simulink model "crazyflie_2015a"  (R2015a)
settings: Solver=ode3  StartTime=0.0  StopTime=30  FixedStep=1/500  MinStep=1e-4  RelTol=1e-3
undefined symbols (not defined in the file): A, B, C, D
libraries: simulink x2
settings Model: NumberOfSteps=250  CovModelRefEnable=off  Creator=mattcollins  LastModifiedBy=mattcollins
settings DataIOCC: SaveFormat=Dataset
settings HardwareCC: ProdBitPerPointer=64  ProdLargestAtomicFloat=Float  ProdIntDivRoundTo=Zero  ProdEndianess=LittleEndian  ProdHWDeviceType=Specified
settings GRTTargetCC: GeneratePreprocessorConditionals=Use local settings

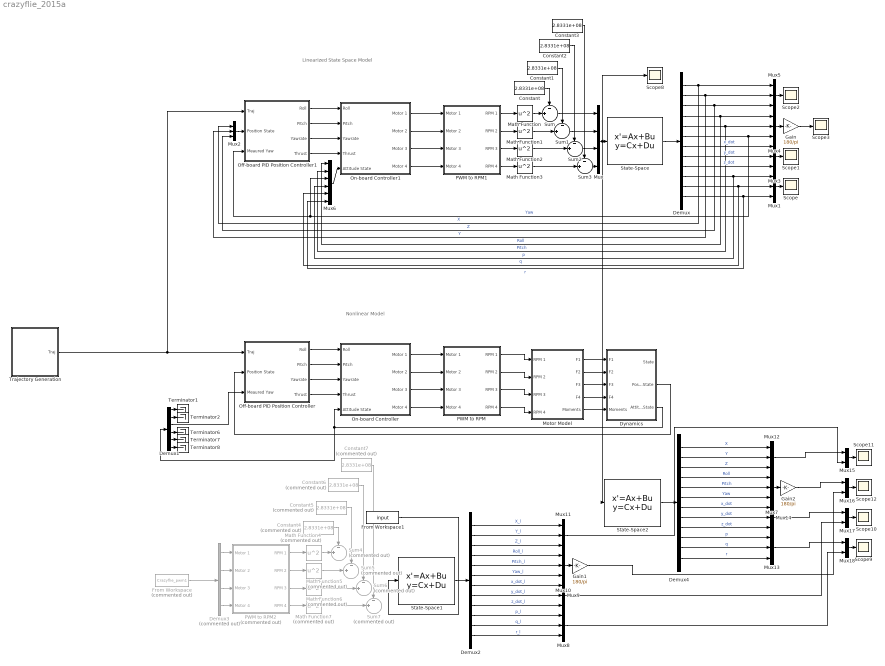
== system crazyflie_2015a ==
  note: Nonlinear Model
  note: Linearized State Space Model
  Constant{,1..3} (4 alike) : Constant  Value=2.8331e+08
  Constant{4..7} (4 alike) : Constant  Commented=on  Value=2.8331e+08
  Demux : Demux  Outputs=12
  Demux1 : Demux  Outputs=6
  Demux2 : Demux  Outputs=12
  Demux3 : Demux  Commented=on
  Demux4 : Demux  Outputs=12
  Dynamics : Subsystem
  From Workspace : FromWorkspace  Commented=on  VariableName=Crazyflie_pwm1  SampleTime=1/500
  From Workspace1 : FromWorkspace  VariableName=input
  Gain : Gain  Gain=180/pi
  Gain1 : Gain  Gain=180/pi
  Gain2 : Gain  Gain=180/pi
  Math Function{,1..3} (4 alike) : Math  Operator=square  SaturateOnIntegerOverflow=on
  Math Function{4..7} (4 alike) : Math  Commented=on  Operator=square  SaturateOnIntegerOverflow=on
  Motor Model : Subsystem
  Mux : Mux
  Mux{1..5,7..14} (13 alike) : Mux  Inputs=3
  Mux{15..18} (4 alike) : Mux  Inputs=2
  Mux6 : Mux  Inputs=6
  Off-board PID Position Controller : Subsystem
  Off-board PID Position Controller1 : Subsystem
  On-board Controller : Subsystem
  On-board Controller1 : Subsystem
  PWM to RPM : Subsystem
  PWM to RPM1 : Subsystem
  PWM to RPM2 : Subsystem  Commented=on
  Scope{,1..3,8..12} (9 alike) : Scope
      Scope settings: TimeRange=auto  ShowLegends=on  MaxDataPoints=5000  SaveToWorkspace=off  YMin=-0.989  YMax=2.74983  SampleTime=-1
      Scope1 settings: TimeRange=auto  ShowLegends=on  MaxDataPoints=5000  SaveToWorkspace=off  SaveName=ScopeData2  YMin=-0.02898  YMax=0.02839  SampleTime=-1
      Scope10 settings: TimeRange=auto  ShowLegends=on  MaxDataPoints=5000  SaveToWorkspace=off  YMin=-5  YMax=5  SampleTime=-1
      Scope11 settings: TimeRange=auto  ShowLegends=on  MaxDataPoints=5000  SaveToWorkspace=off  SaveName=ScopeData2  YMin=-3.50437  YMax=3  SampleTime=-1  DataFormat=Array
      Scope12 settings: TimeRange=auto  ShowLegends=on  MaxDataPoints=5000  SaveToWorkspace=off  SaveName=ScopeData3  YMin=-8.76362  YMax=25  SampleTime=-1  DataFormat=Array
      Scope2 settings: TimeRange=auto  ShowLegends=on  MaxDataPoints=5000  SaveName=Pos_Lin  YMin=-0.86443  YMax=1.76271  SampleTime=-1  DataFormat=Array
      Scope3 settings: TimeRange=auto  ShowLegends=on  MaxDataPoints=5000  SaveName=Att_Lin  YMin=-9.06868  YMax=18.0573  SampleTime=-1  DataFormat=Array
      Scope8 settings: TimeRange=auto  ShowLegends=on  MaxDataPoints=5000  SaveName=input  YMin=-405553.36028  YMax=400152.57445  SampleTime=-1  DataFormat=Array
      Scope9 settings: TimeRange=auto  ShowLegends=on  MaxDataPoints=5000  SaveToWorkspace=off  SaveName=ScopeData4  YMin=-0.989  YMax=2.74983  SampleTime=-1
  State-Space : StateSpace  A=A  B=B  C=C  D=D  X0=[0;0;0;0;0;0;0;0;0;0;0;0]
  State-Space1 : StateSpace  A=A  B=B  C=C  D=D  X0=[0;0;0;0;0;0;0;0;0;0;0;0]
  State-Space2 : StateSpace  A=A  B=B  C=C  D=D  X0=[0;0;0;0;0;0;0;0;0;0;0;0]
  Sum{,1..3} (4 alike) : Sum  Inputs=-|+||
  Sum{4..7} (4 alike) : Sum  Commented=on  Inputs=-|+||
  Terminator{1..2,6..8} (5 alike) : Terminator
  Trajectory Generation : Subsystem
  wires:
  On-board Controller/1(Motor 1) -> PWM to RPM/1(Motor 1)
  On-board Controller/2(Motor 2) -> PWM to RPM/2(Motor 2)
  On-board Controller/3(Motor 3) -> PWM to RPM/3(Motor 3)
  On-board Controller/4(Motor 4) -> PWM to RPM/4(Motor 4)
  PWM to RPM/1(RPM 1) -> Motor Model/1(RPM 1)
  PWM to RPM/2(RPM 2) -> Motor Model/2(RPM 2)
  PWM to RPM/3(RPM 3) -> Motor Model/3(RPM 3)
  PWM to RPM/4(RPM 4) -> Motor Model/4(RPM 4)
  Motor Model/1(F1) -> Dynamics/1(F1)
  Dynamics/3(Attitude State) -> On-board Controller/5(Attitude State), Demux1/1
  Off-board PID Position Controller/1(Roll) -> On-board Controller/1(Roll)
  Off-board PID Position Controller/2(Pitch) -> On-board Controller/2(Pitch)
  Off-board PID Position Controller/3(Yawrate) -> On-board Controller/3(Yawrate)
  Off-board PID Position Controller/4(Thrust) -> On-board Controller/4(Thrust)
  Dynamics/2(Position State) -> Off-board PID Position Controller/2(Position State)
  Motor Model/2(F2) -> Dynamics/2(F2)
  Motor Model/3(F3) -> Dynamics/3(F3)
  Motor Model/4(F4) -> Dynamics/4(F4)
  Motor Model/5(Moments) -> Dynamics/5(Moments)
  Demux1/3 -> Off-board PID Position Controller/3(Meaured Yaw)
  Demux1/1 -> Terminator1/1
  Demux1/2 -> Terminator2/1
  Demux1/4 -> Terminator6/1
  Demux1/5 -> Terminator7/1
  Demux1/6 -> Terminator8/1
  State-Space/1 -> Demux/1
  Demux/10 -> Mux6/4, Mux1/1  "p"
  Demux/11 -> Mux6/5, Mux1/2  "q"
  Demux/12 -> Mux6/6, Mux1/3  "r"
  Mux1/1 -> Scope/1
  Mux3/1 -> Scope1/1
  Demux/7 -> Mux3/1  "x_dot"
  Demux/8 -> Mux3/2  "y_dot"
  Demux/9 -> Mux3/3  "z_dot"
  Demux/4 -> Mux6/1, Mux4/1  "Roll"
  Demux/5 -> Mux6/2, Mux4/2  "Pitch"
  Demux/6 -> Mux6/3, Off-board PID Position Controller1/3(Meaured Yaw), Mux4/3  "Yaw"
  Demux/1 -> Mux2/1, Mux5/1  "X"
  Demux/2 -> Mux2/2, Mux5/2  "Y"
  Demux/3 -> Mux2/3, Mux5/3  "Z"
  Mux4/1 -> Gain/1
  Mux5/1 -> Scope2/1
  PWM to RPM1/1(RPM 1) -> Math Function/1
  PWM to RPM1/2(RPM 2) -> Math Function1/1
  PWM to RPM1/3(RPM 3) -> Math Function2/1
  PWM to RPM1/4(RPM 4) -> Math Function3/1
  On-board Controller1/2(Motor 2) -> PWM to RPM1/2(Motor 2)
  On-board Controller1/3(Motor 3) -> PWM to RPM1/3(Motor 3)
  On-board Controller1/4(Motor 4) -> PWM to RPM1/4(Motor 4)
  Off-board PID Position Controller1/1(Roll) -> On-board Controller1/1(Roll)
  Off-board PID Position Controller1/2(Pitch) -> On-board Controller1/2(Pitch)
  Off-board PID Position Controller1/3(Yawrate) -> On-board Controller1/3(Yawrate)
  Off-board PID Position Controller1/4(Thrust) -> On-board Controller1/4(Thrust)
  Trajectory Generation/1(Traj) -> Off-board PID Position Controller1/1(Traj), Off-board PID Position Controller/1(Traj)
  Mux2/1 -> Off-board PID Position Controller1/2(Position State)
  Mux6/1 -> On-board Controller1/5(Attitude State)
  Gain/1 -> Scope3/1
  Sum/1 -> Mux/1
  Math Function/1 -> Sum/2
  Constant/1 -> Sum/1
  Math Function3/1 -> Sum3/2
  Math Function2/1 -> Sum2/2
  Sum1/1 -> Mux/2
  Math Function1/1 -> Sum1/2
  Sum2/1 -> Mux/3
  Constant1/1 -> Sum1/1
  Constant2/1 -> Sum2/1
  Constant3/1 -> Sum3/1
  State-Space1/1 -> Demux2/1
  Demux2/10 -> Mux8/1  "p_l"
  Demux2/11 -> Mux8/2  "q_l"
  Demux2/12 -> Mux8/3  "r_l"
  Mux8/1 -> Mux18/2
  Mux9/1 -> Mux17/2
  Demux2/7 -> Mux9/1  "x_dot_l"
  Demux2/8 -> Mux9/2  "y_dot_l"
  Demux2/9 -> Mux9/3  "z_dot_l"
  Demux2/4 -> Mux10/1  "Roll_l"
  Demux2/5 -> Mux10/2  "Pitch_l"
  Demux2/6 -> Mux10/3  "Yaw_l"
  Demux2/1 -> Mux11/1  "X_l"
  Demux2/2 -> Mux11/2  "Y_l"
  Demux2/3 -> Mux11/3  "Z_l"
  Mux10/1 -> Gain1/1
  Mux11/1 -> Mux15/2
  PWM to RPM2/1(RPM 1) -> Math Function4/1
  PWM to RPM2/2(RPM 2) -> Math Function5/1
  PWM to RPM2/3(RPM 3) -> Math Function6/1
  PWM to RPM2/4(RPM 4) -> Math Function7/1
  Gain1/1 -> Mux16/2
  Math Function4/1 -> Sum4/2
  Constant4/1 -> Sum4/1
  Math Function7/1 -> Sum7/2
  Math Function6/1 -> Sum6/2
  Math Function5/1 -> Sum5/2
  Constant5/1 -> Sum5/1
  Constant6/1 -> Sum6/1
  Constant7/1 -> Sum7/1
  Demux3/1 -> PWM to RPM2/1(Motor 1)
  Demux3/2 -> PWM to RPM2/2(Motor 2)
  Demux3/3 -> PWM to RPM2/3(Motor 3)
  Demux3/4 -> PWM to RPM2/4(Motor 4)
  From Workspace/1 -> Demux3/1
  Sum3/1 -> Mux/4
  From Workspace1/1 -> State-Space1/1
  State-Space2/1 -> Demux4/1
  Demux4/10 -> Mux13/1  "p"
  Demux4/11 -> Mux13/2  "q"
  Demux4/12 -> Mux13/3  "r"
  Demux4/7 -> Mux14/1  "x_dot"
  Demux4/8 -> Mux14/2  "y_dot"
  Demux4/9 -> Mux14/3  "z_dot"
  Demux4/4 -> Mux7/1  "Roll"
  Demux4/5 -> Mux7/2  "Pitch"
  Demux4/6 -> Mux7/3  "Yaw"
  Demux4/1 -> Mux12/1  "X"
  Demux4/2 -> Mux12/2  "Y"
  Demux4/3 -> Mux12/3  "Z"
  Mux7/1 -> Gain2/1
  Mux/1 -> Scope8/1, State-Space2/1, State-Space/1
  Mux15/1 -> Scope11/1
  Mux16/1 -> Scope12/1
  Mux17/1 -> Scope10/1
  Mux18/1 -> Scope9/1
  Mux12/1 -> Mux15/1
  Gain2/1 -> Mux16/1
  Mux14/1 -> Mux17/1
  Mux13/1 -> Mux18/1
  On-board Controller1/1(Motor 1) -> PWM to RPM1/1(Motor 1)

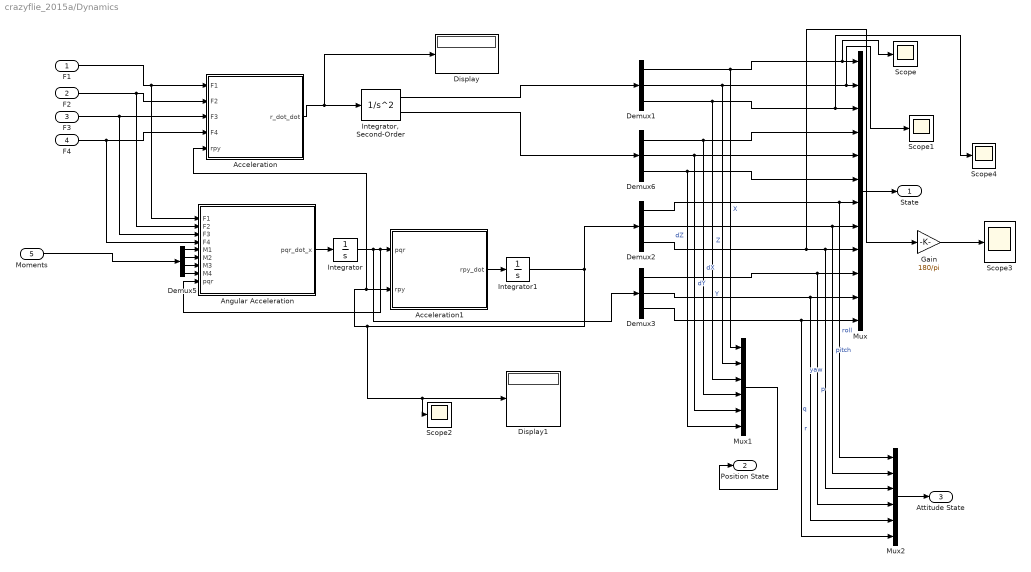
== system crazyflie_2015a/Dynamics ==
  F1 : Inport
  F2 : Inport  Port=2
  F3 : Inport  Port=3
  F4 : Inport  Port=4
  Moments : Inport  Port=5
  Acceleration : MATLAB Function  TreatAsAtomicUnit=on
      settings: PermitHierarchicalResolution=ParametersOnly
  Acceleration1 : MATLAB Function  TreatAsAtomicUnit=on
      settings: PermitHierarchicalResolution=ParametersOnly
  Angular Acceleration : MATLAB Function  TreatAsAtomicUnit=on
      settings: PermitHierarchicalResolution=ParametersOnly
  Demux{1..3,6} (4 alike) : Demux  Outputs=3
  Demux5 : Demux
  Display : Display
  Display1 : Display
  Gain : Gain  Gain=180/pi
  Integrator : Integrator  InitialCondition=[0;0;0]
  "Integrator, Second-Order" : SecondOrderIntegrator  ICX=[0;0;0]  LimitX=on  UpperLimitX=[inf,inf,inf]  LowerLimitX=[-inf,-inf,0]  StateNameX=['x', 'y', 'z']  ICDXDT=[0;0;0]  LimitDXDT=on  UpperLimitDXDT=Inf  LowerLimitDXDT=-Inf  StateNameDXDT=['dx', 'dy', 'dz']
  Integrator1 : Integrator  InitialCondition=[0;0;0]
  Mux : Mux  Inputs=12
  Mux1 : Mux  Inputs=6
  Mux2 : Mux  Inputs=6
  Scope{,1..4} (5 alike) : Scope
      Scope settings: TimeRange=auto  MaxDataPoints=5000  SaveName=x_pos  YMin=-0.15977  YMax=1.43792  SampleTime=-1  DataFormat=Array
      Scope1 settings: TimeRange=auto  MaxDataPoints=5000  SaveName=y_pos  YMin=-0.15994  YMax=1.43948  SampleTime=-1  DataFormat=Array
      Scope2 settings: TimeRange=auto  MaxDataPoints=5000  SaveToWorkspace=off  YMin=-0.00075  YMax=0.00059  SampleTime=-1
      Scope3 settings: TimeRange=auto  MaxDataPoints=5000  SaveName=yaw_pos  YMin=-7.58141  YMax=67.89856  SampleTime=-1  DataFormat=Array
      Scope4 settings: TimeRange=auto  MaxDataPoints=5000  SaveName=z_pos  YMin=0.00000  YMax=1.5  SampleTime=-1  DataFormat=Array
  State : Outport
  Position State : Outport  Port=2
  Attitude State : Outport  Port=3
  wires:
  Demux2/1 -> Mux2/1, Mux/7  "roll"
  Demux2/2 -> Mux2/2, Mux/8  "pitch"
  Demux2/3 -> Gain/1, Mux2/3, Mux/9  "yaw"
  Demux3/1 -> Mux2/4, Mux/10  "p"
  Demux3/2 -> Mux2/5, Mux/11  "q"
  Demux3/3 -> Mux2/6, Mux/12  "r"
  Mux/1 -> State/1
  Mux1/1 -> Position State/1
  Mux2/1 -> Attitude State/1
  Demux5/1 -> Angular Acceleration/5(M1)
  Demux5/2 -> Angular Acceleration/6(M2)
  Demux5/3 -> Angular Acceleration/7(M3)
  Demux5/4 -> Angular Acceleration/8(M4)
  Angular Acceleration/1(pqr_dot_x) -> Integrator/1
  Integrator/1 -> Demux3/1, Angular Acceleration/9(pqr), Acceleration1/1(pqr)
  Acceleration1/1(rpy_dot) -> Integrator1/1
  Integrator1/1 -> Demux2/1, Scope2/1, Display1/1, Acceleration/5(rpy), Acceleration1/2(rpy)
  Acceleration/1(r_dot_dot) -> Display/1, "Integrator, Second-Order"/1
  "Integrator, Second-Order"/1 -> Demux1/1
  "Integrator, Second-Order"/2 -> Demux6/1
  Demux1/1 -> Mux1/1, Scope/1, Mux/1  "X"
  Demux1/2 -> Mux1/2, Scope1/1, Mux/2  "Y"
  Demux1/3 -> Mux1/3, Scope4/1, Mux/3  "Z"
  Demux6/1 -> Mux1/4, Mux/4  "dX"
  Demux6/2 -> Mux1/5, Mux/5  "dY"
  Demux6/3 -> Mux1/6, Mux/6  "dZ"
  Moments/1 -> Demux5/1
  F2/1 -> Angular Acceleration/2(F2), Acceleration/2(F2)
  F3/1 -> Angular Acceleration/3(F3), Acceleration/3(F3)
  F4/1 -> Angular Acceleration/4(F4), Acceleration/4(F4)
  F1/1 -> Angular Acceleration/1(F1), Acceleration/1(F1)
  Gain/1 -> Scope3/1

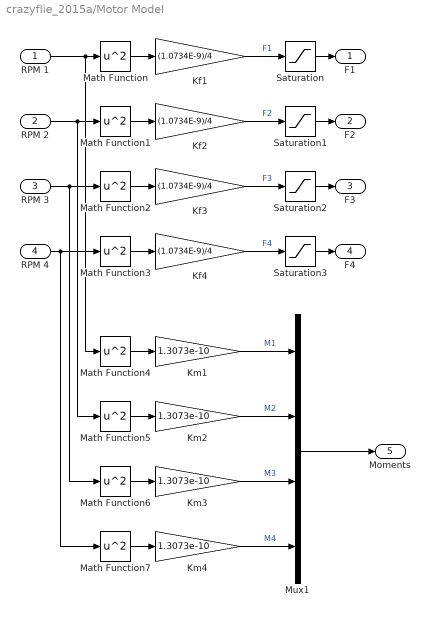
== system crazyflie_2015a/Motor Model ==
  RPM 1 : Inport
  RPM 2 : Inport  Port=2
  RPM 3 : Inport  Port=3
  RPM 4 : Inport  Port=4
  Kf{1..4} (4 alike) : Gain  Gain=(1.0734E-9)/4
  Km{1..4} (4 alike) : Gain  Gain=1.3073e-10
  Math Function{,1..7} (8 alike) : Math  Operator=square  SaturateOnIntegerOverflow=on
  Mux1 : Mux
  Saturation{,1..3} (4 alike) : Saturate  UpperLimit=.2  LowerLimit=0
  F1 : Outport
  F2 : Outport  Port=2
  F3 : Outport  Port=3
  F4 : Outport  Port=4
  Moments : Outport  Port=5
  wires:
  RPM 4/1 -> Math Function7/1, Math Function3/1
  RPM 3/1 -> Math Function6/1, Math Function2/1
  RPM 2/1 -> Math Function5/1, Math Function1/1
  RPM 1/1 -> Math Function4/1, Math Function/1
  Math Function/1 -> Kf1/1
  Math Function1/1 -> Kf2/1
  Math Function2/1 -> Kf3/1
  Math Function3/1 -> Kf4/1
  Kf3/1 -> Saturation2/1  "F3"
  Math Function4/1 -> Km1/1
  Math Function5/1 -> Km2/1
  Math Function6/1 -> Km3/1
  Math Function7/1 -> Km4/1
  Km4/1 -> Mux1/4  "M4"
  Km3/1 -> Mux1/3  "M3"
  Km2/1 -> Mux1/2  "M2"
  Km1/1 -> Mux1/1  "M1"
  Mux1/1 -> Moments/1
  Kf2/1 -> Saturation1/1  "F2"
  Kf1/1 -> Saturation/1  "F1"
  Kf4/1 -> Saturation3/1  "F4"
  Saturation/1 -> F1/1
  Saturation1/1 -> F2/1
  Saturation2/1 -> F3/1
  Saturation3/1 -> F4/1

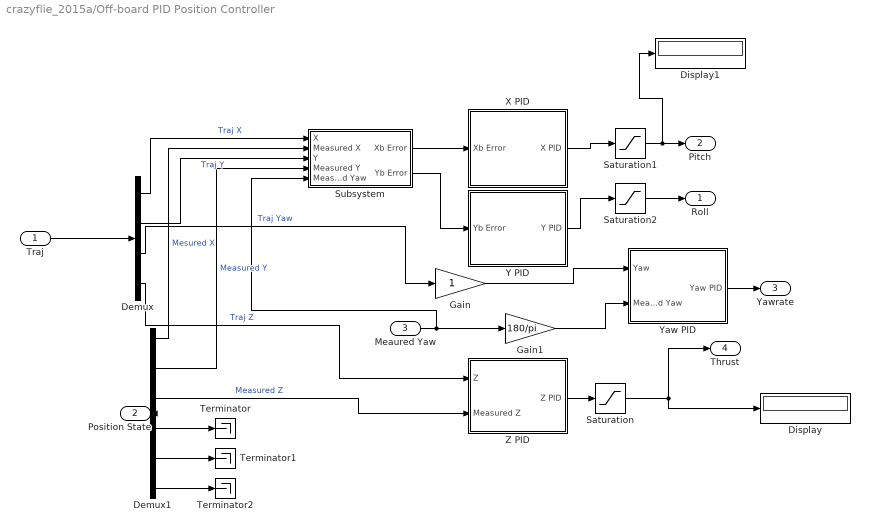
== system crazyflie_2015a/Off-board PID Position Controller ==
  Traj : Inport
  Position State : Inport  Port=2
  Meaured Yaw : Inport  Port=3
  Demux : Demux
  Demux1 : Demux  Outputs=6
  Display : Display
  Display1 : Display
  Gain : Gain
  Gain1 : Gain  Gain=180/pi
  Saturation : Saturate  UpperLimit=60000  LowerLimit=1000
  Saturation1 : Saturate  UpperLimit=30  LowerLimit=-30
  Saturation2 : Saturate  UpperLimit=30  LowerLimit=-30
  Subsystem : Subsystem
  Terminator : Terminator
  Terminator1 : Terminator
  Terminator2 : Terminator
  X PID : Subsystem
  Y PID : Subsystem
  Yaw PID : Subsystem
  Z PID : Subsystem
  Roll : Outport
  Pitch : Outport  Port=2
  Yawrate : Outport  Port=3
  Thrust : Outport  Port=4
  wires:
  Traj/1 -> Demux/1
  X PID/1(X PID) -> Saturation1/1
  Demux/4 -> Z PID/1(Z)  "Traj Z"
  Demux/3 -> Gain/1  "Traj Yaw"
  Position State/1 -> Demux1/1
  Demux1/4 -> Terminator/1
  Demux1/5 -> Terminator1/1
  Demux1/6 -> Terminator2/1
  Demux1/3 -> Z PID/2(Measured Z)  "Measured Z"
  Y PID/1(Y PID) -> Saturation2/1
  Z PID/1(Z PID) -> Saturation/1
  Saturation/1 -> Display/1, Thrust/1
  Saturation1/1 -> Pitch/1, Display1/1
  Saturation2/1 -> Roll/1
  Yaw PID/1(Yaw PID) -> Yawrate/1
  Meaured Yaw/1 -> Subsystem/5(Measured Yaw), Gain1/1
  Gain/1 -> Yaw PID/1(Yaw)
  Gain1/1 -> Yaw PID/2(Measured Yaw)
  Subsystem/1(Xb Error) -> X PID/1(Xb Error)
  Subsystem/2(Yb Error) -> Y PID/1(Yb Error)
  Demux/1 -> Subsystem/1(X)  "Traj X"
  Demux/2 -> Subsystem/3(Y)  "Traj Y"
  Demux1/1 -> Subsystem/2(Measured X)  "Mesured X"
  Demux1/2 -> Subsystem/4(Measured Y)  "Measured Y"

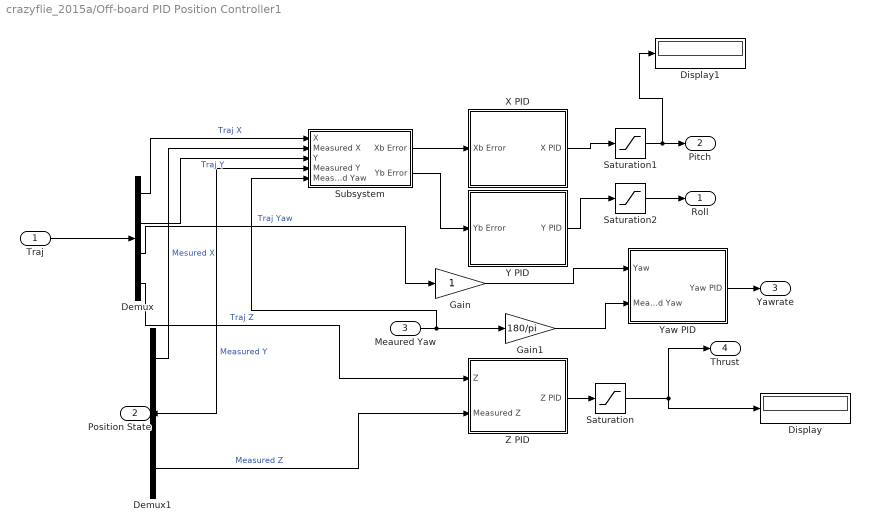
== system crazyflie_2015a/Off-board PID Position Controller1 ==
  Traj : Inport
  Position State : Inport  Port=2
  Meaured Yaw : Inport  Port=3
  Demux : Demux
  Demux1 : Demux  Outputs=3
  Display : Display
  Display1 : Display
  Gain : Gain
  Gain1 : Gain  Gain=180/pi
  Saturation : Saturate  UpperLimit=60000  LowerLimit=1000
  Saturation1 : Saturate  UpperLimit=30  LowerLimit=-30
  Saturation2 : Saturate  UpperLimit=30  LowerLimit=-30
  Subsystem : Subsystem
  X PID : Subsystem
  Y PID : Subsystem
  Yaw PID : Subsystem
  Z PID : Subsystem
  Roll : Outport
  Pitch : Outport  Port=2
  Yawrate : Outport  Port=3
  Thrust : Outport  Port=4
  wires:
  Traj/1 -> Demux/1
  X PID/1(X PID) -> Saturation1/1
  Demux/4 -> Z PID/1(Z)  "Traj Z"
  Demux/3 -> Gain/1  "Traj Yaw"
  Position State/1 -> Demux1/1
  Demux1/3 -> Z PID/2(Measured Z)  "Measured Z"
  Y PID/1(Y PID) -> Saturation2/1
  Z PID/1(Z PID) -> Saturation/1
  Saturation/1 -> Display/1, Thrust/1
  Saturation1/1 -> Pitch/1, Display1/1
  Saturation2/1 -> Roll/1
  Yaw PID/1(Yaw PID) -> Yawrate/1
  Meaured Yaw/1 -> Subsystem/5(Measured Yaw), Gain1/1
  Gain/1 -> Yaw PID/1(Yaw)
  Gain1/1 -> Yaw PID/2(Measured Yaw)
  Subsystem/1(Xb Error) -> X PID/1(Xb Error)
  Subsystem/2(Yb Error) -> Y PID/1(Yb Error)
  Demux/1 -> Subsystem/1(X)  "Traj X"
  Demux/2 -> Subsystem/3(Y)  "Traj Y"
  Demux1/1 -> Subsystem/2(Measured X)  "Mesured X"
  Demux1/2 -> Subsystem/4(Measured Y)  "Measured Y"

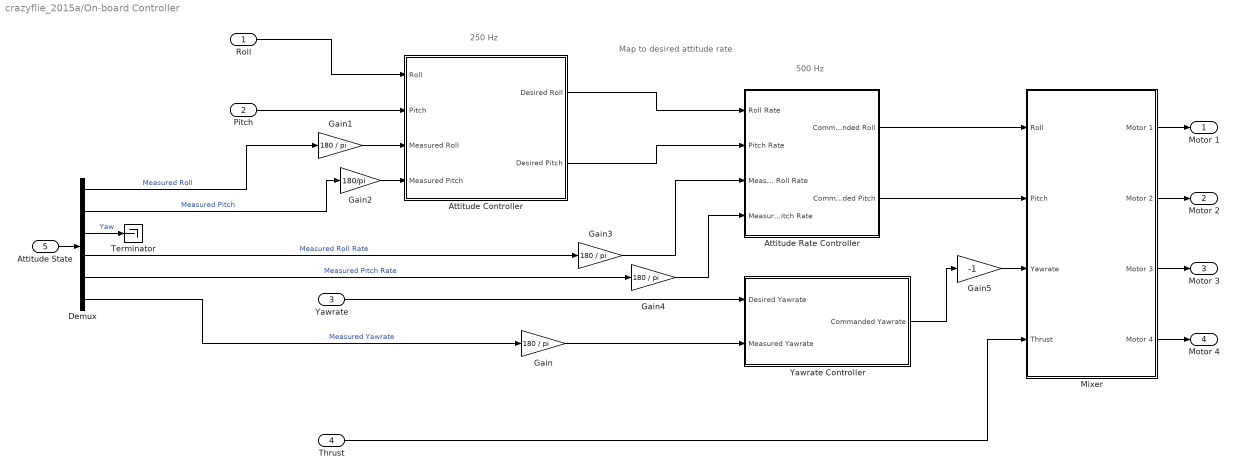
== system crazyflie_2015a/On-board Controller ==
  note: 500 Hz
  note: Map to desired
      | attitude rate
  note: 250 Hz
  Roll : Inport
  Pitch : Inport  Port=2
  Yawrate : Inport  Port=3
  Thrust : Inport  Port=4
  Attitude State : Inport  Port=5
  "Attitude Controller " : Subsystem
  Attitude Rate Controller : Subsystem
  Demux : Demux  Outputs=6
  Gain{,1,3..4} (4 alike) : Gain  Gain=180 / pi
  Gain2 : Gain  Gain=180/pi
  Gain5 : Gain  Gain=-1
  Mixer : Subsystem
  Terminator : Terminator
  "Yawrate Controller " : Subsystem
  Motor 1 : Outport
  Motor 2 : Outport  Port=2
  Motor 3 : Outport  Port=3
  Motor 4 : Outport  Port=4
  wires:
  Yawrate/1 -> "Yawrate Controller "/1(Desired Yawrate)
  Attitude Rate Controller/1(Commanded Roll) -> Mixer/1(Roll)
  Attitude Rate Controller/2(Commanded Pitch) -> Mixer/2(Pitch)
  "Yawrate Controller "/1(Commanded Yawrate) -> Gain5/1
  Thrust/1 -> Mixer/4(Thrust)
  Mixer/1(Motor 1) -> Motor 1/1
  Mixer/2(Motor 2) -> Motor 2/1
  Mixer/3(Motor 3) -> Motor 3/1
  Mixer/4(Motor 4) -> Motor 4/1
  Attitude State/1 -> Demux/1
  Demux/1 -> Gain1/1  "Measured Roll"
  Demux/2 -> Gain2/1  "Measured Pitch"
  Demux/4 -> Gain3/1  "Measured Roll Rate"
  Demux/5 -> Gain4/1  "Measured Pitch Rate"
  Demux/3 -> Terminator/1  "Yaw"
  Roll/1 -> "Attitude Controller "/1(Roll)
  Pitch/1 -> "Attitude Controller "/2(Pitch)
  "Attitude Controller "/1(Desired Roll) -> Attitude Rate Controller/1(Roll Rate)
  "Attitude Controller "/2("Desired Pitch ") -> Attitude Rate Controller/2(Pitch Rate)
  Gain/1 -> "Yawrate Controller "/2(Measured Yawrate)
  Demux/6 -> Gain/1  "Measured Yawrate"
  Gain1/1 -> "Attitude Controller "/3(Measured Roll)
  Gain2/1 -> "Attitude Controller "/4(Measured Pitch)
  Gain3/1 -> Attitude Rate Controller/3(Measured Roll Rate)
  Gain4/1 -> Attitude Rate Controller/4(Measured Pitch Rate)
  Gain5/1 -> Mixer/3(Yawrate)

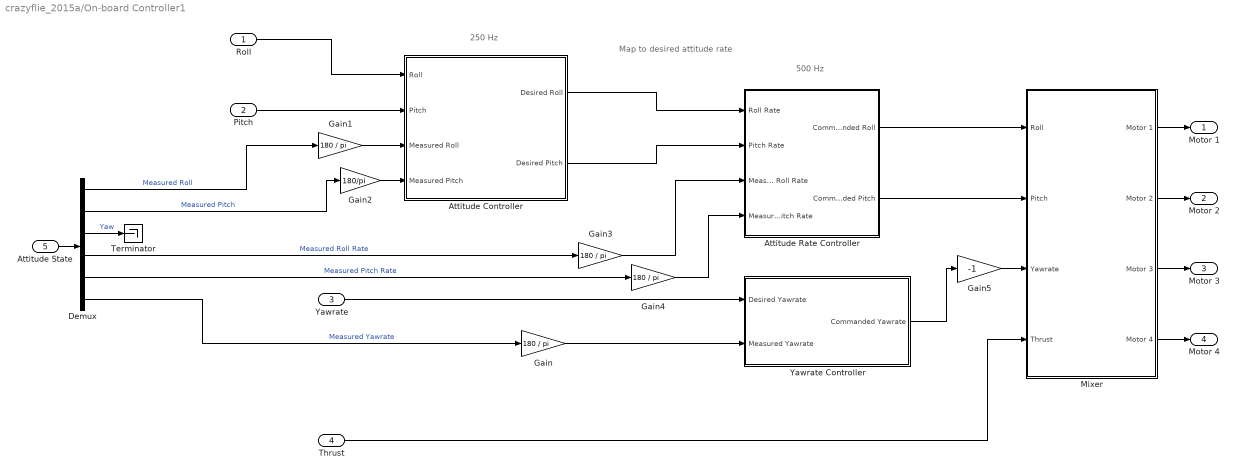
== system crazyflie_2015a/On-board Controller1 ==
  note: 500 Hz
  note: Map to desired
      | attitude rate
  note: 250 Hz
  Roll : Inport
  Pitch : Inport  Port=2
  Yawrate : Inport  Port=3
  Thrust : Inport  Port=4
  Attitude State : Inport  Port=5
  "Attitude Controller " : Subsystem
  Attitude Rate Controller : Subsystem
  Demux : Demux  Outputs=6
  Gain{,1,3..4} (4 alike) : Gain  Gain=180 / pi
  Gain2 : Gain  Gain=180/pi
  Gain5 : Gain  Gain=-1
  Mixer : Subsystem
  Terminator : Terminator
  "Yawrate Controller " : Subsystem
  Motor 1 : Outport
  Motor 2 : Outport  Port=2
  Motor 3 : Outport  Port=3
  Motor 4 : Outport  Port=4
  wires:
  Yawrate/1 -> "Yawrate Controller "/1(Desired Yawrate)
  Attitude Rate Controller/1(Commanded Roll) -> Mixer/1(Roll)
  Attitude Rate Controller/2(Commanded Pitch) -> Mixer/2(Pitch)
  "Yawrate Controller "/1(Commanded Yawrate) -> Gain5/1
  Thrust/1 -> Mixer/4(Thrust)
  Mixer/1(Motor 1) -> Motor 1/1
  Mixer/2(Motor 2) -> Motor 2/1
  Mixer/3(Motor 3) -> Motor 3/1
  Mixer/4(Motor 4) -> Motor 4/1
  Attitude State/1 -> Demux/1
  Demux/1 -> Gain1/1  "Measured Roll"
  Demux/2 -> Gain2/1  "Measured Pitch"
  Demux/4 -> Gain3/1  "Measured Roll Rate"
  Demux/5 -> Gain4/1  "Measured Pitch Rate"
  Demux/3 -> Terminator/1  "Yaw"
  Roll/1 -> "Attitude Controller "/1(Roll)
  Pitch/1 -> "Attitude Controller "/2(Pitch)
  "Attitude Controller "/1(Desired Roll) -> Attitude Rate Controller/1(Roll Rate)
  "Attitude Controller "/2("Desired Pitch ") -> Attitude Rate Controller/2(Pitch Rate)
  Gain/1 -> "Yawrate Controller "/2(Measured Yawrate)
  Demux/6 -> Gain/1  "Measured Yawrate"
  Gain1/1 -> "Attitude Controller "/3(Measured Roll)
  Gain2/1 -> "Attitude Controller "/4(Measured Pitch)
  Gain3/1 -> Attitude Rate Controller/3(Measured Roll Rate)
  Gain4/1 -> Attitude Rate Controller/4(Measured Pitch Rate)
  Gain5/1 -> Mixer/3(Yawrate)

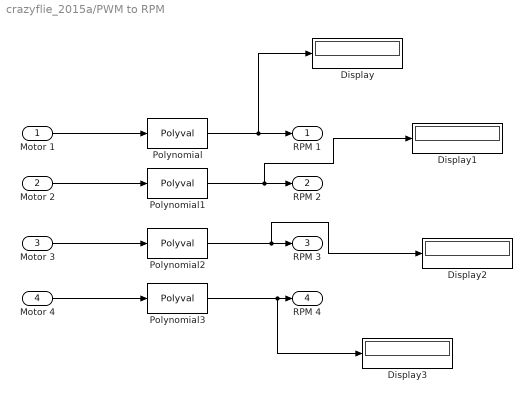
== system crazyflie_2015a/PWM to RPM ==
  Motor 1 : Inport
  Motor 2 : Inport  Port=2
  Motor 3 : Inport  Port=3
  Motor 4 : Inport  Port=4
  Display{,1..3} (4 alike) : Display
  Polynomial{,1..3} (4 alike) : Polyval  Coefs=[1.6809E-19 -3.0288E-14 2.0739E-09 -6.7596E-05 1.3515E+00 0]
  RPM 1 : Outport
  RPM 2 : Outport  Port=2
  RPM 3 : Outport  Port=3
  RPM 4 : Outport  Port=4
  wires:
  Motor 1/1 -> Polynomial/1
  Polynomial/1 -> Display/1, RPM 1/1
  Motor 2/1 -> Polynomial1/1
  Polynomial1/1 -> Display1/1, RPM 2/1
  Motor 3/1 -> Polynomial2/1
  Polynomial2/1 -> Display2/1, RPM 3/1
  Motor 4/1 -> Polynomial3/1
  Polynomial3/1 -> Display3/1, RPM 4/1

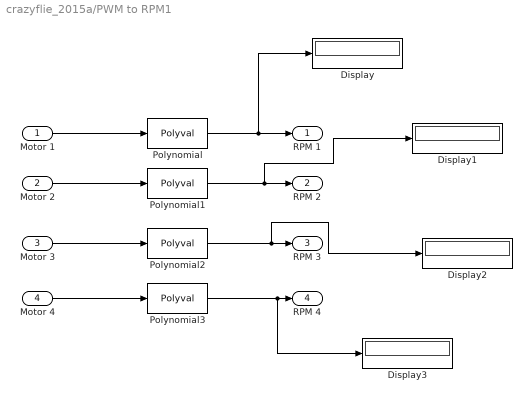
== system crazyflie_2015a/PWM to RPM1 ==
  Motor 1 : Inport
  Motor 2 : Inport  Port=2
  Motor 3 : Inport  Port=3
  Motor 4 : Inport  Port=4
  Display{,1..3} (4 alike) : Display
  Polynomial{,1..3} (4 alike) : Polyval  Coefs=[1.6809E-19 -3.0288E-14 2.0739E-09 -6.7596E-05 1.3515E+00 0]
  RPM 1 : Outport
  RPM 2 : Outport  Port=2
  RPM 3 : Outport  Port=3
  RPM 4 : Outport  Port=4
  wires:
  Motor 1/1 -> Polynomial/1
  Polynomial/1 -> Display/1, RPM 1/1
  Motor 2/1 -> Polynomial1/1
  Polynomial1/1 -> Display1/1, RPM 2/1
  Motor 3/1 -> Polynomial2/1
  Polynomial2/1 -> Display2/1, RPM 3/1
  Motor 4/1 -> Polynomial3/1
  Polynomial3/1 -> Display3/1, RPM 4/1

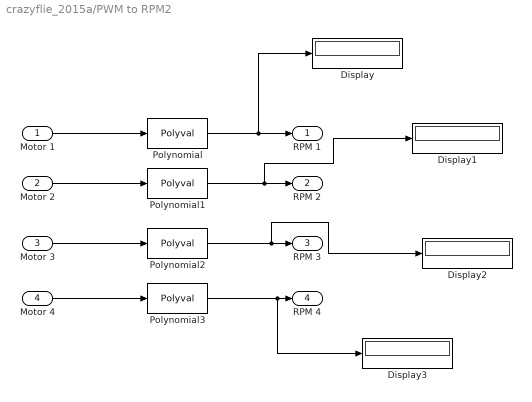
== system crazyflie_2015a/PWM to RPM2 ==
  Motor 1 : Inport
  Motor 2 : Inport  Port=2
  Motor 3 : Inport  Port=3
  Motor 4 : Inport  Port=4
  Display{,1..3} (4 alike) : Display
  Polynomial{,1..3} (4 alike) : Polyval  Coefs=[1.6809E-19 -3.0288E-14 2.0739E-09 -6.7596E-05 1.3515E+00 0]
  RPM 1 : Outport
  RPM 2 : Outport  Port=2
  RPM 3 : Outport  Port=3
  RPM 4 : Outport  Port=4
  wires:
  Motor 1/1 -> Polynomial/1
  Polynomial/1 -> Display/1, RPM 1/1
  Motor 2/1 -> Polynomial1/1
  Polynomial1/1 -> Display1/1, RPM 2/1
  Motor 3/1 -> Polynomial2/1
  Polynomial2/1 -> Display2/1, RPM 3/1
  Motor 4/1 -> Polynomial3/1
  Polynomial3/1 -> Display3/1, RPM 4/1

== system crazyflie_2015a/Trajectory Generation ==
  Mux : Mux
  Ramp : simulink/Sources/Ramp  slope=.05  start=0  X0=0
  Ramp1 : simulink/Sources/Ramp  slope=50  start=5  X0=0
  Scope{,1..3} (4 alike) : Scope
      Scope settings: TimeRange=auto  MaxDataPoints=5000  SaveName=z_ref  YMin=-0.125  YMax=1.125  SampleTime=-1  DataFormat=Array
      Scope1 settings: TimeRange=auto  MaxDataPoints=5000  SaveName=y_ref  YMin=-0.125  YMax=1.125  SampleTime=-1  DataFormat=Array
      Scope2 settings: TimeRange=auto  MaxDataPoints=5000  SaveName=x_ref  YMin=-0.125  YMax=1.125  SampleTime=-1  DataFormat=Array
      Scope3 settings: TimeRange=auto  MaxDataPoints=5000  SaveName=yaw_ref  YMin=-7.5  YMax=67.5  SampleTime=-1  DataFormat=Array
  Sine Wave1 : Sin  Amplitude=.5  Frequency=pi/10  Phase=-pi/2  SampleTime=0
  Sine Wave2 : Sin  Amplitude=.5  Frequency=pi/10  SampleTime=0
  Step : Step  Time=10  SampleTime=0
  Step1 : Step  SampleTime=0
  Step2 : Step  Time=5  SampleTime=0
  Step3 : Step  Time=15  After=60  SampleTime=0
  Traj : Outport
  wires:
  Mux/1 -> Traj/1
  Sine Wave1/1 -> Scope2/1, Mux/1
  Sine Wave2/1 -> Scope1/1, Mux/2
  Ramp/1 -> Scope/1, Mux/4
  Ramp1/1 -> Mux/3, Scope3/1

== system crazyflie_2015a/Off-board PID Position Controller/Subsystem ==
  X : Inport
  Measured X : Inport  Port=2
  Y : Inport  Port=3
  Measured Y : Inport  Port=4
  Measured Yaw : Inport  Port=5
  Demux : Demux  Outputs=2
  MATLAB Function : MATLAB Function  TreatAsAtomicUnit=on
      settings: PermitHierarchicalResolution=ParametersOnly
  Mux : Mux  Inputs=2
  Product : Product  Multiplication=Matrix(*)
  Sum : Sum  Inputs=|+-
  Sum1 : Sum  Inputs=|+-
  Xb Error : Outport
  Yb Error : Outport  Port=2
  wires:
  X/1 -> Sum/1
  Measured X/1 -> Sum/2
  Y/1 -> Sum1/1
  Measured Y/1 -> Sum1/2
  Sum/1 -> Mux/1
  Sum1/1 -> Mux/2
  Product/1 -> Demux/1
  Demux/1 -> Xb Error/1
  Demux/2 -> Yb Error/1
  Measured Yaw/1 -> MATLAB Function/1(yaw)
  MATLAB Function/1(R_m) -> Product/1
  Mux/1 -> Product/2  "Xw Error"

== system crazyflie_2015a/Off-board PID Position Controller/X PID ==
  Xb Error : Inport
  Derivative : Derivative
  Integrator : Integrator
  Kd : Gain  Gain=10
  Ki : Gain  Gain=4
  Kp : Gain  Gain=18
  Saturation : Saturate  UpperLimit=.2  LowerLimit=-.2
  Sum3 : Sum  Inputs=+++
  X PID : Outport
  wires:
  Xb Error/1 -> Derivative/1, Integrator/1, Kp/1
  Kp/1 -> Sum3/1
  Kd/1 -> Sum3/3
  Sum3/1 -> X PID/1
  Ki/1 -> Sum3/2
  Saturation/1 -> Ki/1
  Integrator/1 -> Saturation/1
  Derivative/1 -> Kd/1

== system crazyflie_2015a/Off-board PID Position Controller/Y PID ==
  Yb Error : Inport
  Derivative : Derivative
  Integrator : Integrator
  Kd : Gain  Gain=10
  Ki : Gain  Gain=4
  Kp : Gain  Gain=18
  Saturation : Saturate  UpperLimit=.2  LowerLimit=-.2
  Sum3 : Sum  Inputs=+++
  Y PID : Outport
  wires:
  Yb Error/1 -> Derivative/1, Integrator/1, Kp/1
  Kp/1 -> Sum3/1
  Kd/1 -> Sum3/3
  Sum3/1 -> Y PID/1
  Ki/1 -> Sum3/2
  Saturation/1 -> Ki/1
  Integrator/1 -> Saturation/1
  Derivative/1 -> Kd/1

== system crazyflie_2015a/Off-board PID Position Controller/Yaw PID ==
  Yaw : Inport
  Measured Yaw : Inport  Port=2
  Derivative : Derivative
  Integrator : Integrator
  Kd : Gain
  Ki : Gain  Gain=0
  Kp : Gain  Gain=3
  Saturation : Saturate  UpperLimit=.2  LowerLimit=-.2
  Sum2 : Sum  Inputs=|+-
  Sum3 : Sum  Inputs=+++
  Yaw PID : Outport
  wires:
  Yaw/1 -> Sum2/1
  Measured Yaw/1 -> Sum2/2
  Sum2/1 -> Derivative/1, Integrator/1, Kp/1
  Kp/1 -> Sum3/1
  Kd/1 -> Sum3/3
  Sum3/1 -> Yaw PID/1
  Ki/1 -> Sum3/2
  Saturation/1 -> Ki/1
  Integrator/1 -> Saturation/1
  Derivative/1 -> Kd/1

== system crazyflie_2015a/Off-board PID Position Controller/Z PID ==
  Z : Inport
  Measured Z : Inport  Port=2
  Derivative : Derivative
  Integrator : Integrator
  Kd : Gain  Gain=40000
  Ki : Gain  Gain=10000
  Kp : Gain  Gain=50000
  PID Limit : Saturate  UpperLimit=25000  LowerLimit=-25000
  Saturation : Saturate  UpperLimit=10  LowerLimit=-10
  Sum : Sum  Inputs=|++
  Sum2 : Sum  Inputs=|+-
  Sum3 : Sum  Inputs=+++
  Thrust Base : Constant  Value=35125.3
  Z PID : Outport
  wires:
  Sum2/1 -> Integrator/1, Derivative/1, Kp/1
  Kp/1 -> Sum3/1
  Kd/1 -> Sum3/3
  Ki/1 -> Sum3/2
  Saturation/1 -> Ki/1
  Thrust Base/1 -> Sum/2
  Sum/1 -> Z PID/1
  Sum3/1 -> PID Limit/1
  PID Limit/1 -> Sum/1
  Z/1 -> Sum2/1
  Measured Z/1 -> Sum2/2
  Integrator/1 -> Saturation/1
  Derivative/1 -> Kd/1

== system crazyflie_2015a/Off-board PID Position Controller1/Subsystem ==
  X : Inport
  Measured X : Inport  Port=2
  Y : Inport  Port=3
  Measured Y : Inport  Port=4
  Measured Yaw : Inport  Port=5
  Demux : Demux  Outputs=2
  MATLAB Function : MATLAB Function  TreatAsAtomicUnit=on
      settings: PermitHierarchicalResolution=ParametersOnly
  Mux : Mux  Inputs=2
  Product : Product  Multiplication=Matrix(*)
  Sum : Sum  Inputs=|+-
  Sum1 : Sum  Inputs=|+-
  Xb Error : Outport
  Yb Error : Outport  Port=2
  wires:
  X/1 -> Sum/1
  Measured X/1 -> Sum/2
  Y/1 -> Sum1/1
  Measured Y/1 -> Sum1/2
  Sum/1 -> Mux/1
  Sum1/1 -> Mux/2
  Product/1 -> Demux/1
  Demux/1 -> Xb Error/1
  Demux/2 -> Yb Error/1
  Measured Yaw/1 -> MATLAB Function/1(yaw)
  MATLAB Function/1(R_m) -> Product/1
  Mux/1 -> Product/2  "Xw Error"

== system crazyflie_2015a/Off-board PID Position Controller1/X PID ==
  Xb Error : Inport
  Derivative : Derivative
  Integrator : Integrator
  Kd : Gain  Gain=10
  Ki : Gain  Gain=4
  Kp : Gain  Gain=18
  Saturation : Saturate  UpperLimit=.2  LowerLimit=-.2
  Sum3 : Sum  Inputs=+++
  X PID : Outport
  wires:
  Xb Error/1 -> Derivative/1, Integrator/1, Kp/1
  Kp/1 -> Sum3/1
  Kd/1 -> Sum3/3
  Sum3/1 -> X PID/1
  Ki/1 -> Sum3/2
  Saturation/1 -> Ki/1
  Integrator/1 -> Saturation/1
  Derivative/1 -> Kd/1

== system crazyflie_2015a/Off-board PID Position Controller1/Y PID ==
  Yb Error : Inport
  Derivative : Derivative
  Integrator : Integrator
  Kd : Gain  Gain=10
  Ki : Gain  Gain=4
  Kp : Gain  Gain=18
  Saturation : Saturate  UpperLimit=.2  LowerLimit=-.2
  Sum3 : Sum  Inputs=+++
  Y PID : Outport
  wires:
  Yb Error/1 -> Derivative/1, Integrator/1, Kp/1
  Kp/1 -> Sum3/1
  Kd/1 -> Sum3/3
  Sum3/1 -> Y PID/1
  Ki/1 -> Sum3/2
  Saturation/1 -> Ki/1
  Integrator/1 -> Saturation/1
  Derivative/1 -> Kd/1

== system crazyflie_2015a/Off-board PID Position Controller1/Yaw PID ==
  Yaw : Inport
  Measured Yaw : Inport  Port=2
  Derivative : Derivative
  Integrator : Integrator
  Kd : Gain
  Ki : Gain  Gain=0
  Kp : Gain  Gain=3
  Saturation : Saturate  UpperLimit=.2  LowerLimit=-.2
  Sum2 : Sum  Inputs=|+-
  Sum3 : Sum  Inputs=+++
  Yaw PID : Outport
  wires:
  Yaw/1 -> Sum2/1
  Measured Yaw/1 -> Sum2/2
  Sum2/1 -> Derivative/1, Integrator/1, Kp/1
  Kp/1 -> Sum3/1
  Kd/1 -> Sum3/3
  Sum3/1 -> Yaw PID/1
  Ki/1 -> Sum3/2
  Saturation/1 -> Ki/1
  Integrator/1 -> Saturation/1
  Derivative/1 -> Kd/1

== system crazyflie_2015a/Off-board PID Position Controller1/Z PID ==
  Z : Inport
  Measured Z : Inport  Port=2
  Derivative : Derivative
  Integrator : Integrator
  Kd : Gain  Gain=40000
  Ki : Gain  Gain=10000
  Kp : Gain  Gain=50000
  PID Limit : Saturate  UpperLimit=25000  LowerLimit=-25000
  Saturation : Saturate  UpperLimit=10  LowerLimit=-10
  Sum : Sum  Inputs=|++
  Sum2 : Sum  Inputs=|+-
  Sum3 : Sum  Inputs=+++
  Thrust Base : Constant  Value=35125.3
  Z PID : Outport
  wires:
  Sum2/1 -> Integrator/1, Derivative/1, Kp/1
  Kp/1 -> Sum3/1
  Kd/1 -> Sum3/3
  Ki/1 -> Sum3/2
  Saturation/1 -> Ki/1
  Thrust Base/1 -> Sum/2
  Sum/1 -> Z PID/1
  Sum3/1 -> PID Limit/1
  PID Limit/1 -> Sum/1
  Z/1 -> Sum2/1
  Measured Z/1 -> Sum2/2
  Integrator/1 -> Saturation/1
  Derivative/1 -> Kd/1

== system crazyflie_2015a/On-board Controller/Attitude Controller  ==
  Roll : Inport
  Pitch : Inport  Port=2
  Measured Roll : Inport  Port=3
  Measured Pitch : Inport  Port=4
  Pitch PID : Subsystem
  Roll PID : Subsystem
  Desired Roll : Outport
  "Desired Pitch " : Outport  Port=2
  wires:
  Pitch/1 -> Pitch PID/1(Pitch)
  Measured Pitch/1 -> Pitch PID/2(Measured Pitch)
  Pitch PID/1(Pitch PID) -> "Desired Pitch "/1
  Measured Roll/1 -> Roll PID/2(Measured Roll)
  Roll/1 -> Roll PID/1(Roll)
  Roll PID/1(Roll PID) -> Desired Roll/1

== system crazyflie_2015a/On-board Controller/Attitude Rate Controller ==
  Roll Rate : Inport
  Pitch Rate : Inport  Port=2
  Measured Roll Rate : Inport  Port=3
  Measured Pitch Rate : Inport  Port=4
  Pitch Rate PID : Subsystem
  Roll Rate PID : Subsystem
  Saturation : Saturate  UpperLimit=2^15  LowerLimit=-2^15
  Saturation1 : Saturate  UpperLimit=2^15  LowerLimit=-2^15
  Commanded Roll : Outport
  Commanded Pitch : Outport  Port=2
  wires:
  Roll Rate/1 -> Roll Rate PID/1(Roll Rate)
  Measured Roll Rate/1 -> Roll Rate PID/2(Measured Roll Rate)
  Pitch Rate/1 -> Pitch Rate PID/1(Pitch Ratel)
  Measured Pitch Rate/1 -> Pitch Rate PID/2(Measured Pitch Rate)
  Roll Rate PID/1(Roll Rate PID) -> Saturation/1
  Pitch Rate PID/1(Pitch Rate PID) -> Saturation1/1
  Saturation/1 -> Commanded Roll/1
  Saturation1/1 -> Commanded Pitch/1

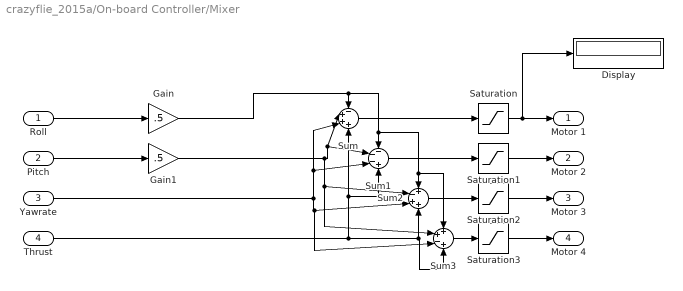
== system crazyflie_2015a/On-board Controller/Mixer ==
  Roll : Inport
  Pitch : Inport  Port=2
  Yawrate : Inport  Port=3
  Thrust : Inport  Port=4
  Display : Display
  Gain : Gain  Gain=.5
  Gain1 : Gain  Gain=.5
  Saturation{,1..3} (4 alike) : Saturate  UpperLimit=2^16  LowerLimit=0
  Sum : Sum  Inputs=-+++
  Sum1 : Sum  Inputs=---+
  Sum2 : Sum  Inputs=+-++
  Sum3 : Sum  Inputs=++-+
  Motor 1 : Outport
  Motor 2 : Outport  Port=2
  Motor 3 : Outport  Port=3
  Motor 4 : Outport  Port=4
  wires:
  Roll/1 -> Gain/1
  Pitch/1 -> Gain1/1
  Yawrate/1 -> Sum1/3, Sum/3, Sum3/3, Sum2/3
  Thrust/1 -> Sum2/4, Sum3/4, Sum1/4, Sum/4
  Sum/1 -> Saturation/1
  Sum2/1 -> Saturation2/1
  Sum3/1 -> Saturation3/1
  Sum1/1 -> Saturation1/1
  Gain/1 -> Sum3/1, Sum2/1, Sum1/1, Sum/1
  Gain1/1 -> Sum3/2, Sum2/2, Sum1/2, Sum/2
  Saturation1/1 -> Motor 2/1
  Saturation2/1 -> Motor 3/1
  Saturation3/1 -> Motor 4/1
  Saturation/1 -> Display/1, Motor 1/1

== system crazyflie_2015a/On-board Controller/Yawrate Controller  ==
  Desired Yawrate : Inport
  Measured Yawrate : Inport  Port=2
  Yawrate PID : Subsystem
  Commanded Yawrate : Outport
  wires:
  Yawrate PID/1(Yawrate PID) -> Commanded Yawrate/1
  Desired Yawrate/1 -> Yawrate PID/1(Yawrate)
  Measured Yawrate/1 -> Yawrate PID/2(Measured Yawrate)

== system crazyflie_2015a/On-board Controller1/Attitude Controller  ==
  Roll : Inport
  Pitch : Inport  Port=2
  Measured Roll : Inport  Port=3
  Measured Pitch : Inport  Port=4
  Pitch PID : Subsystem
  Roll PID : Subsystem
  Desired Roll : Outport
  "Desired Pitch " : Outport  Port=2
  wires:
  Pitch/1 -> Pitch PID/1(Pitch)
  Measured Pitch/1 -> Pitch PID/2(Measured Pitch)
  Pitch PID/1(Pitch PID) -> "Desired Pitch "/1
  Measured Roll/1 -> Roll PID/2(Measured Roll)
  Roll/1 -> Roll PID/1(Roll)
  Roll PID/1(Roll PID) -> Desired Roll/1

== system crazyflie_2015a/On-board Controller1/Attitude Rate Controller ==
  Roll Rate : Inport
  Pitch Rate : Inport  Port=2
  Measured Roll Rate : Inport  Port=3
  Measured Pitch Rate : Inport  Port=4
  Pitch Rate PID : Subsystem
  Roll Rate PID : Subsystem
  Saturation : Saturate  UpperLimit=2^15  LowerLimit=-2^15
  Saturation1 : Saturate  UpperLimit=2^15  LowerLimit=-2^15
  Commanded Roll : Outport
  Commanded Pitch : Outport  Port=2
  wires:
  Roll Rate/1 -> Roll Rate PID/1(Roll Rate)
  Measured Roll Rate/1 -> Roll Rate PID/2(Measured Roll Rate)
  Pitch Rate/1 -> Pitch Rate PID/1(Pitch Ratel)
  Measured Pitch Rate/1 -> Pitch Rate PID/2(Measured Pitch Rate)
  Roll Rate PID/1(Roll Rate PID) -> Saturation/1
  Pitch Rate PID/1(Pitch Rate PID) -> Saturation1/1
  Saturation/1 -> Commanded Roll/1
  Saturation1/1 -> Commanded Pitch/1

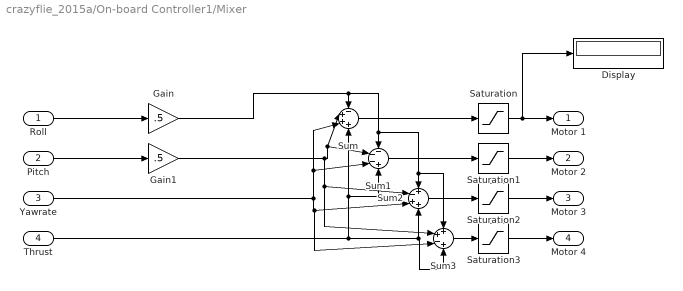
== system crazyflie_2015a/On-board Controller1/Mixer ==
  Roll : Inport
  Pitch : Inport  Port=2
  Yawrate : Inport  Port=3
  Thrust : Inport  Port=4
  Display : Display
  Gain : Gain  Gain=.5
  Gain1 : Gain  Gain=.5
  Saturation{,1..3} (4 alike) : Saturate  UpperLimit=2^16  LowerLimit=0
  Sum : Sum  Inputs=-+++
  Sum1 : Sum  Inputs=---+
  Sum2 : Sum  Inputs=+-++
  Sum3 : Sum  Inputs=++-+
  Motor 1 : Outport
  Motor 2 : Outport  Port=2
  Motor 3 : Outport  Port=3
  Motor 4 : Outport  Port=4
  wires:
  Roll/1 -> Gain/1
  Pitch/1 -> Gain1/1
  Yawrate/1 -> Sum1/3, Sum/3, Sum3/3, Sum2/3
  Thrust/1 -> Sum2/4, Sum3/4, Sum1/4, Sum/4
  Sum/1 -> Saturation/1
  Sum2/1 -> Saturation2/1
  Sum3/1 -> Saturation3/1
  Sum1/1 -> Saturation1/1
  Gain/1 -> Sum3/1, Sum2/1, Sum1/1, Sum/1
  Gain1/1 -> Sum3/2, Sum2/2, Sum1/2, Sum/2
  Saturation1/1 -> Motor 2/1
  Saturation2/1 -> Motor 3/1
  Saturation3/1 -> Motor 4/1
  Saturation/1 -> Display/1, Motor 1/1

== system crazyflie_2015a/On-board Controller1/Yawrate Controller  ==
  Desired Yawrate : Inport
  Measured Yawrate : Inport  Port=2
  Yawrate PID : Subsystem
  Commanded Yawrate : Outport
  wires:
  Yawrate PID/1(Yawrate PID) -> Commanded Yawrate/1
  Desired Yawrate/1 -> Yawrate PID/1(Yawrate)
  Measured Yawrate/1 -> Yawrate PID/2(Measured Yawrate)

== system crazyflie_2015a/On-board Controller/Attitude Controller /Pitch PID ==
  Pitch : Inport
  Measured Pitch : Inport  Port=2
  Derivative : Derivative
  Integrator Limited : Integrator  LimitOutput=on  UpperSaturationLimit=20  LowerSaturationLimit=-20
  Kd1 : Gain  Gain=0
  Ki1 : Gain  Gain=4
  Kp1 : Gain  Gain=10
  Sum1 : Sum  Inputs=|+-
  Sum6 : Sum  Inputs=+++
  Pitch PID : Outport
  wires:
  Pitch/1 -> Sum1/1
  Measured Pitch/1 -> Sum1/2
  Sum1/1 -> Integrator Limited/1, Derivative/1, Kp1/1
  Kp1/1 -> Sum6/1
  Kd1/1 -> Sum6/3
  Sum6/1 -> Pitch PID/1
  Ki1/1 -> Sum6/2
  Derivative/1 -> Kd1/1
  Integrator Limited/1 -> Ki1/1

== system crazyflie_2015a/On-board Controller/Attitude Controller /Roll PID ==
  Roll : Inport
  Measured Roll : Inport  Port=2
  Derivative : Derivative
  Integrator Limited : Integrator  LimitOutput=on  UpperSaturationLimit=20  LowerSaturationLimit=-20
  Kd : Gain  Gain=0
  Ki : Gain  Gain=4
  Kp : Gain  Gain=10
  Sum2 : Sum  Inputs=|+-
  Sum3 : Sum  Inputs=+++
  Roll PID : Outport
  wires:
  Roll/1 -> Sum2/1
  Measured Roll/1 -> Sum2/2
  Sum2/1 -> Integrator Limited/1, Derivative/1, Kp/1
  Kp/1 -> Sum3/1
  Kd/1 -> Sum3/3
  Sum3/1 -> Roll PID/1
  Ki/1 -> Sum3/2
  Derivative/1 -> Kd/1
  Integrator Limited/1 -> Ki/1

== system crazyflie_2015a/On-board Controller/Attitude Rate Controller/Pitch Rate PID ==
  Pitch Ratel : Inport
  Measured Pitch Rate : Inport  Port=2
  Derivative : Derivative
  Integrator Limited : Integrator  LimitOutput=on  UpperSaturationLimit=33.3  LowerSaturationLimit=-33.3
  Kd : Gain  Gain=2.5
  Ki : Gain  Gain=500
  Kp : Gain  Gain=250
  Sum2 : Sum  Inputs=|+-
  Sum3 : Sum  Inputs=+++
  Pitch Rate PID : Outport
  wires:
  Pitch Ratel/1 -> Sum2/1
  Measured Pitch Rate/1 -> Sum2/2
  Sum2/1 -> Integrator Limited/1, Derivative/1, Kp/1
  Kp/1 -> Sum3/1
  Kd/1 -> Sum3/3
  Sum3/1 -> Pitch Rate PID/1
  Ki/1 -> Sum3/2
  Integrator Limited/1 -> Ki/1
  Derivative/1 -> Kd/1

== system crazyflie_2015a/On-board Controller/Attitude Rate Controller/Roll Rate PID ==
  Roll Rate : Inport
  Measured Roll Rate : Inport  Port=2
  Derivative : Derivative
  Integrator : Integrator
  Kd : Gain  Gain=2.5
  Ki : Gain  Gain=500
  Kp : Gain  Gain=250
  Saturation : Saturate  UpperLimit=33.3  LowerLimit=-33.3
  Sum2 : Sum  Inputs=|+-
  Sum3 : Sum  Inputs=+++
  Roll Rate PID : Outport
  wires:
  Roll Rate/1 -> Sum2/1
  Measured Roll Rate/1 -> Sum2/2
  Sum2/1 -> Derivative/1, Integrator/1, Kp/1
  Kp/1 -> Sum3/1
  Kd/1 -> Sum3/3
  Sum3/1 -> Roll Rate PID/1
  Ki/1 -> Sum3/2
  Saturation/1 -> Ki/1
  Integrator/1 -> Saturation/1
  Derivative/1 -> Kd/1

== system crazyflie_2015a/On-board Controller/Yawrate Controller /Yawrate PID ==
  Yawrate : Inport
  Measured Yawrate : Inport  Port=2
  Derivative : Derivative
  Integrator : Integrator
  Kd : Gain  Gain=0
  Ki : Gain  Gain=16.7
  Kp : Gain  Gain=70
  Saturation : Saturate  UpperLimit=166.7  LowerLimit=-166.7
  Sum : Sum  Inputs=|+-
  Sum1 : Sum  Inputs=+++
  Yawrate PID : Outport
  wires:
  Yawrate/1 -> Sum/1
  Measured Yawrate/1 -> Sum/2
  Sum/1 -> Integrator/1, Derivative/1, Kp/1
  Kp/1 -> Sum1/1
  Kd/1 -> Sum1/3
  Sum1/1 -> Yawrate PID/1
  Ki/1 -> Sum1/2
  Saturation/1 -> Ki/1
  Derivative/1 -> Kd/1
  Integrator/1 -> Saturation/1

== system crazyflie_2015a/On-board Controller1/Attitude Controller /Pitch PID ==
  Pitch : Inport
  Measured Pitch : Inport  Port=2
  Derivative : Derivative
  Integrator Limited : Integrator  LimitOutput=on  UpperSaturationLimit=20  LowerSaturationLimit=-20
  Kd1 : Gain  Gain=0
  Ki1 : Gain  Gain=4
  Kp1 : Gain  Gain=10
  Sum1 : Sum  Inputs=|+-
  Sum6 : Sum  Inputs=+++
  Pitch PID : Outport
  wires:
  Pitch/1 -> Sum1/1
  Measured Pitch/1 -> Sum1/2
  Sum1/1 -> Integrator Limited/1, Derivative/1, Kp1/1
  Kp1/1 -> Sum6/1
  Kd1/1 -> Sum6/3
  Sum6/1 -> Pitch PID/1
  Ki1/1 -> Sum6/2
  Derivative/1 -> Kd1/1
  Integrator Limited/1 -> Ki1/1

== system crazyflie_2015a/On-board Controller1/Attitude Controller /Roll PID ==
  Roll : Inport
  Measured Roll : Inport  Port=2
  Derivative : Derivative
  Integrator Limited : Integrator  LimitOutput=on  UpperSaturationLimit=20  LowerSaturationLimit=-20
  Kd : Gain  Gain=0
  Ki : Gain  Gain=4
  Kp : Gain  Gain=10
  Sum2 : Sum  Inputs=|+-
  Sum3 : Sum  Inputs=+++
  Roll PID : Outport
  wires:
  Roll/1 -> Sum2/1
  Measured Roll/1 -> Sum2/2
  Sum2/1 -> Integrator Limited/1, Derivative/1, Kp/1
  Kp/1 -> Sum3/1
  Kd/1 -> Sum3/3
  Sum3/1 -> Roll PID/1
  Ki/1 -> Sum3/2
  Derivative/1 -> Kd/1
  Integrator Limited/1 -> Ki/1

== system crazyflie_2015a/On-board Controller1/Attitude Rate Controller/Pitch Rate PID ==
  Pitch Ratel : Inport
  Measured Pitch Rate : Inport  Port=2
  Derivative : Derivative
  Integrator Limited : Integrator  LimitOutput=on  UpperSaturationLimit=33.3  LowerSaturationLimit=-33.3
  Kd : Gain  Gain=2.5
  Ki : Gain  Gain=500
  Kp : Gain  Gain=250
  Sum2 : Sum  Inputs=|+-
  Sum3 : Sum  Inputs=+++
  Pitch Rate PID : Outport
  wires:
  Pitch Ratel/1 -> Sum2/1
  Measured Pitch Rate/1 -> Sum2/2
  Sum2/1 -> Integrator Limited/1, Derivative/1, Kp/1
  Kp/1 -> Sum3/1
  Kd/1 -> Sum3/3
  Sum3/1 -> Pitch Rate PID/1
  Ki/1 -> Sum3/2
  Integrator Limited/1 -> Ki/1
  Derivative/1 -> Kd/1

== system crazyflie_2015a/On-board Controller1/Attitude Rate Controller/Roll Rate PID ==
  Roll Rate : Inport
  Measured Roll Rate : Inport  Port=2
  Derivative : Derivative
  Integrator : Integrator
  Kd : Gain  Gain=2.5
  Ki : Gain  Gain=500
  Kp : Gain  Gain=250
  Saturation : Saturate  UpperLimit=33.3  LowerLimit=-33.3
  Sum2 : Sum  Inputs=|+-
  Sum3 : Sum  Inputs=+++
  Roll Rate PID : Outport
  wires:
  Roll Rate/1 -> Sum2/1
  Measured Roll Rate/1 -> Sum2/2
  Sum2/1 -> Derivative/1, Integrator/1, Kp/1
  Kp/1 -> Sum3/1
  Kd/1 -> Sum3/3
  Sum3/1 -> Roll Rate PID/1
  Ki/1 -> Sum3/2
  Saturation/1 -> Ki/1
  Integrator/1 -> Saturation/1
  Derivative/1 -> Kd/1

== system crazyflie_2015a/On-board Controller1/Yawrate Controller /Yawrate PID ==
  Yawrate : Inport
  Measured Yawrate : Inport  Port=2
  Derivative : Derivative
  Integrator : Integrator
  Kd : Gain  Gain=0
  Ki : Gain  Gain=16.7
  Kp : Gain  Gain=70
  Saturation : Saturate  UpperLimit=166.7  LowerLimit=-166.7
  Sum : Sum  Inputs=|+-
  Sum1 : Sum  Inputs=+++
  Yawrate PID : Outport
  wires:
  Yawrate/1 -> Sum/1
  Measured Yawrate/1 -> Sum/2
  Sum/1 -> Integrator/1, Derivative/1, Kp/1
  Kp/1 -> Sum1/1
  Kd/1 -> Sum1/3
  Sum1/1 -> Yawrate PID/1
  Ki/1 -> Sum1/2
  Saturation/1 -> Ki/1
  Derivative/1 -> Kd/1
  Integrator/1 -> Saturation/1

== matlab function crazyflie_2015a/Dynamics/Angular Acceleration ==
  data: F1 input double [0..1]; pqr_dot_x output; F2 input double [0..1]; F3 input double [0..1]; F4 input double [0..1]; M1 input; M2 input; M3 input; M4 input; pqr input
function pqr_dot_x = Crazyflie_ang(F1,F2,F3,F4,M1,M2,M3,M4,pqr)
%#codegen
pqr_dot_x = zeros(3,1);
L = 0.0455;
Ixx = 2.3951E-05;
Iyy = 2.3951E-05;
Izz = 3.2347E-05;
I_matrix = diag([Ixx Iyy Izz]);

Eq1 = [L/sqrt(2)*(F3+F4-F1-F2); ...
      L/sqrt(2)*(F1+F4-F2-F3); ...
      -M1+M2-M3+M4];
Eq2 = cross(pqr, I_matrix*pqr);
  
pqr_dot = inv(I_matrix)*(Eq1 - Eq2);


pqr_dot_x = pqr_dot;

== matlab function crazyflie_2015a/Dynamics/Acceleration ==
  data: F1 input double; F2 input; F3 input; F4 input; r_dot_dot output; rpy input
function r_dot_dot = Crazyflie_accel(F1,F2,F3,F4,rpy)
%#codegen
r_dot_dot = zeros(3,1);
m = 0.031;
g = [0;0;-9.81];

Wrb = [cos(rpy(3))*cos(rpy(2))+sin(rpy(1))*sin(rpy(2))*sin(rpy(3)) -cos(rpy(1))*sin(rpy(3)) cos(rpy(3))*sin(rpy(2))-cos(rpy(2))*sin(rpy(1))*sin(rpy(3)); ...
       cos(rpy(2))*sin(rpy(3))-cos(rpy(3))*sin(rpy(1))*sin(rpy(2)) cos(rpy(1))*cos(rpy(3)) sin(rpy(3))*sin(rpy(2))+cos(rpy(3))*cos(rpy(2))*sin(rpy(1)); ...
       -cos(rpy(1))*sin(rpy(2)) -sin(rpy(1)) cos(rpy(1))*cos(rpy(2))];  
r_dot_dot = g + 1/m * Wrb*[0;0;sum([F1 F2 F3 F4])];

== matlab function crazyflie_2015a/Dynamics/Acceleration1 ==
  data: pqr input; rpy_dot output; rpy input
function rpy_dot = Crazyflie_rpy(pqr, rpy)
%#codegen
rpy_dot = zeros(3,1);
Wrb = [cos(rpy(2)) 0 -cos(rpy(1))*sin(rpy(2)); ...
       0 1 sin(rpy(1)); ...
       sin(rpy(2)) 0 cos(rpy(1))*cos(rpy(2))];
  
rpy_dot = Wrb\pqr;

== matlab function crazyflie_2015a/Off-board PID Position Controller/Subsystem/MATLAB Function ==
  data: yaw input; R_m output
function R_m = Error_transform(yaw)
%#codegen

R_m = [cos(yaw) sin(yaw); -sin(yaw) cos(yaw)];

== matlab function crazyflie_2015a/Off-board PID Position Controller1/Subsystem/MATLAB Function ==
  data: yaw input; R_m output
function R_m = Error_transform(yaw)
%#codegen

R_m = eye(2);
%[cos(yaw) sin(yaw); -sin(yaw) cos(yaw)];
